simulink model "tamtoplayicidevre"  (R2013a)
settings: Solver=ode45  StartTime=0.0  StopTime=10.0  RelTol=1e-3
settings Model: Creator=Lenovo  LastModifiedBy=Lenovo

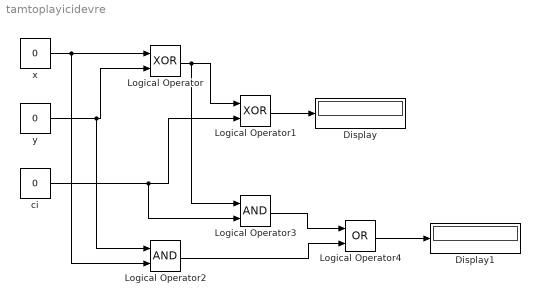
== system tamtoplayicidevre ==
  Display : Display
  Display1 : Display
  Logical Operator : Logic  Operator=XOR  AllPortsSameDT=off  OutDataTypeStr=boolean
  Logical Operator1 : Logic  Operator=XOR  AllPortsSameDT=off  OutDataTypeStr=boolean
  Logical Operator2 : Logic  AllPortsSameDT=off  OutDataTypeStr=boolean
  Logical Operator3 : Logic  AllPortsSameDT=off  OutDataTypeStr=boolean
  Logical Operator4 : Logic  Operator=OR  AllPortsSameDT=off  OutDataTypeStr=boolean
  ci : Constant  Value=0
  x : Constant  Value=0
  y : Constant  Value=0
  wires:
  x/1 -> Logical Operator2/2, Logical Operator/1
  y/1 -> Logical Operator2/1, Logical Operator/2
  Logical Operator/1 -> Logical Operator3/1, Logical Operator1/1
  Logical Operator1/1 -> Display/1
  ci/1 -> Logical Operator3/2, Logical Operator1/2
  Logical Operator2/1 -> Logical Operator4/2
  Logical Operator3/1 -> Logical Operator4/1
  Logical Operator4/1 -> Display1/1
